simulink model "Gantry_sim1"  (R2024b)
settings: Solver=VariableStepAuto  StartTime=0.0  StopTime=5  RelTol=1e-6
undefined symbols (not defined in the file): g1, g2, wl1, wl2, wnotch, wr1, wr2, zl1, zl2, znotch, zr1, zr2
settings Model: Creator=olgai  LastModifiedBy=olgai

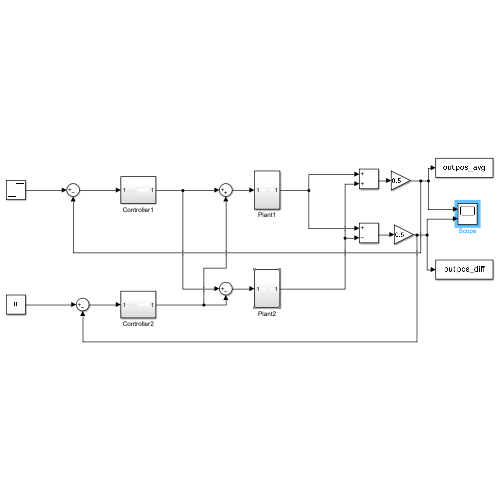
[thumbnail: Simulink's stored preview of the top-level diagram]
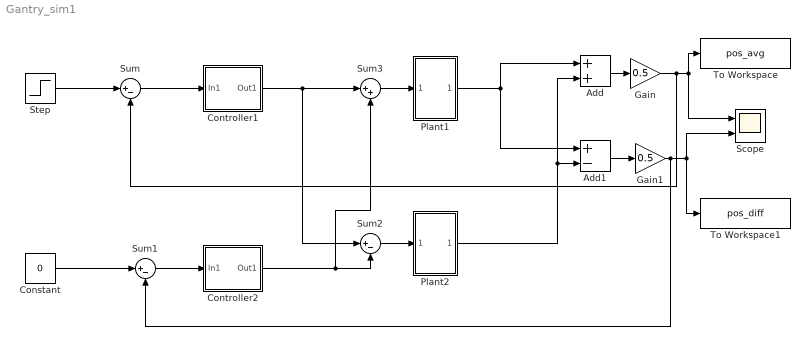
== system Gantry_sim1 ==
  Add : Sum
  Add1 : Sum  Inputs=+-
  Constant : Constant  Value=0
  Controller1 : Subsystem
  Controller2 : Subsystem
  Gain : Gain  Gain=0.5
  Gain1 : Gain  Gain=0.5
  Plant1 : Subsystem
  Plant2 : Subsystem
  Scope : Scope  NumInputPorts=2
  Step : Step  SampleTime=0
  Sum : Sum  Inputs=|+-
  Sum1 : Sum  Inputs=|+-
  Sum2 : Sum  Inputs=|+-
  Sum3 : Sum  Inputs=|++
  To Workspace : ToWorkspace  VariableName=pos_avg  SaveFormat=Timeseries  SampleTime=-1
  To Workspace1 : ToWorkspace  VariableName=pos_diff  SaveFormat=Timeseries  SampleTime=-1
  wires:
  Step/1 -> Sum/1
  Plant1/1(Out1) -> Add1/1, Add/1
  Plant2/1(Out1) -> Add/2, Add1/2
  Add/1 -> Gain/1
  Add1/1 -> Gain1/1
  Gain/1 -> Sum/2, Scope/1, To Workspace/1
  Gain1/1 -> Sum1/2, To Workspace1/1, Scope/2
  Sum/1 -> Controller1/1(In1)
  Controller1/1(Out1) -> Sum2/1, Sum3/1
  Constant/1 -> Sum1/1
  Sum1/1 -> Controller2/1(In1)
  Sum2/1 -> Plant2/1(In1)
  Controller2/1(Out1) -> Sum3/2, Sum2/2
  Sum3/1 -> Plant1/1(In1)

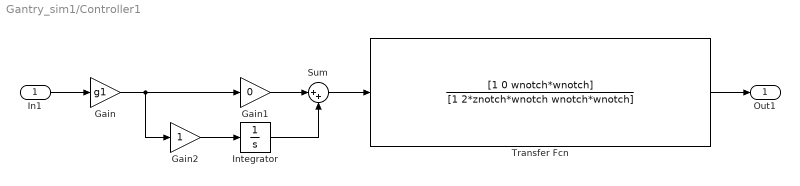
== system Gantry_sim1/Controller1 ==
  In1 : Inport
  Gain : Gain  Gain=g1
  Gain1 : Gain  Gain=0
  Gain2 : Gain
  Integrator : Integrator
  Sum : Sum  Inputs=|++
  Transfer Fcn : TransferFcn  Numerator=[1 0 wnotch*wnotch]  Denominator=[1 2*znotch*wnotch wnotch*wnotch]
  Out1 : Outport
  wires:
  In1/1 -> Gain/1
  Integrator/1 -> Sum/2
  Gain/1 -> Gain1/1, Gain2/1
  Sum/1 -> Transfer Fcn/1
  Gain1/1 -> Sum/1
  Gain2/1 -> Integrator/1
  Transfer Fcn/1 -> Out1/1

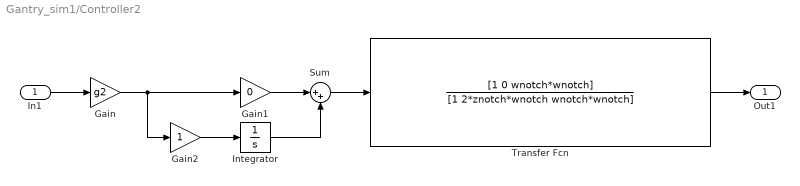
== system Gantry_sim1/Controller2 ==
  In1 : Inport
  Gain : Gain  Gain=g2
  Gain1 : Gain  Gain=0
  Gain2 : Gain
  Integrator : Integrator
  Sum : Sum  Inputs=|++
  Transfer Fcn : TransferFcn  Numerator=[1 0 wnotch*wnotch]  Denominator=[1 2*znotch*wnotch wnotch*wnotch]
  Out1 : Outport
  wires:
  In1/1 -> Gain/1
  Integrator/1 -> Sum/2
  Gain/1 -> Gain1/1, Gain2/1
  Sum/1 -> Transfer Fcn/1
  Gain1/1 -> Sum/1
  Gain2/1 -> Integrator/1
  Transfer Fcn/1 -> Out1/1

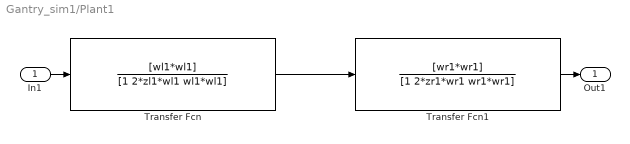
== system Gantry_sim1/Plant1 ==
  In1 : Inport
  Transfer Fcn : TransferFcn  Numerator=[wl1*wl1]  Denominator=[1 2*zl1*wl1 wl1*wl1]
  Transfer Fcn1 : TransferFcn  Numerator=[wr1*wr1]  Denominator=[1 2*zr1*wr1 wr1*wr1]
  Out1 : Outport
  wires:
  Transfer Fcn/1 -> Transfer Fcn1/1
  In1/1 -> Transfer Fcn/1
  Transfer Fcn1/1 -> Out1/1

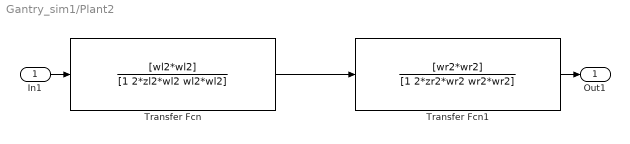
== system Gantry_sim1/Plant2 ==
  In1 : Inport
  Transfer Fcn : TransferFcn  Numerator=[wl2*wl2]  Denominator=[1 2*zl2*wl2 wl2*wl2]
  Transfer Fcn1 : TransferFcn  Numerator=[wr2*wr2]  Denominator=[1 2*zr2*wr2 wr2*wr2]
  Out1 : Outport
  wires:
  Transfer Fcn/1 -> Transfer Fcn1/1
  In1/1 -> Transfer Fcn/1
  Transfer Fcn1/1 -> Out1/1
